simulink model "PubIfDecisionTOS_MDL"  (R2020b)
settings: configuration reference "DspaceConfig" (kept outside this file)
PostLoadFcn:
  | if any(exist('dsrtsu_mdlpostloadfcn', 'file') ~= 0), dsrtsu_mdlpostloadfcn('Execute', bdroot); end
InitFcn:
  | , if any(exist('dsmpb_private', 'file') ~= 0), dsmpb_private('dsmpb_mdlclblib', 'Init', bdroot); end,
undefined symbols (not defined in the file or in its folder): C_TOS_ACCEgoRAxletoFbumplength_m, C_TOS_ACCTargetFront_Flag, C_TOS_AEBJAPedObjDxThre_Val, C_TOS_AEBJAPedObjDyThre_Val, C_TOS_AEBJATargetSize_Val, C_TOS_AEBJAVehObjDxThre_Val, C_TOS_AEBJAVehObjDyThre_Val, C_TOS_AEBJuncPedTargetSize_Val, C_TOS_AEBLatObjDxThre_Val, C_TOS_AEBLatPedDyThre_Val, C_TOS_AEBLatTargetSize_Val, C_TOS_AEBLongTargetInEgoFront_Flag, C_TOS_axAbsGround_Parameter, C_TOS_CameraConfirmedFlag, C_TOS_CNsubjWidth, C_TOS_CurrentLaneCoreMinWidth_Val, C_TOS_CutInProb_Val_Zero, C_TOS_CutOutProb_Val_Zero, C_TOS_D2R_Val, C_TOS_DefaultValueObjectToCenterLine_dy, C_TOS_EgoCarWidth_Val, C_TOS_EgoDxRefPoint_m, C_TOS_EgoRAxletoFbumplength_m, C_TOS_HalfWidthVehicle_Con, C_TOS_HWA_CurrentLaneFlag, C_TOS_HWA_LeftLaneFlag, C_TOS_HWA_MovingDir_Vaild, C_TOS_HWA_MovState_Vaild, C_TOS_HWA_RightLaneFlag, C_TOS_LaneLineCourseErrorFront, C_TOS_LaneLineCourseErrorRear, C_TOS_MotorbikeDefaultWidth_m, C_TOS_NumberOfEffectiveTargets, C_TOS_Obj_Age_Val, C_TOS_Objdx_Constraint_Val, C_TOS_ObjectDefaultWidth_m, C_TOS_ObjInCurrentLane_Val, C_TOS_ObjInCurrentLaneValid, C_TOS_ObjInLeftLaneValid, C_TOS_ObjInRightLaneValid, C_TOS_ObjNotInCurrentLane_Val, C_TOS_ObjNotREElementType, C_TOS_ObjPredictDis_dy_ConstantVal_Zeros, C_TOS_ObjToCenterLine_ConstantVal_Zeros, C_TOS_OFMObjIDInvilad_Val, C_TOS_PIL_LatDisCons_Val_zero, C_TOS_PIL_ObjectCutInFlag_b, C_TOS_PIL_ObjectCutOutFlag_b, C_TOS_PIL_ObjLaneProb_al_Val, C_TOS_PP_ObjFusType_FC_Confirm_b, C_TOS_PP_ObjFusType_FC_FR_Confirm_b, C_TOS_PP_ObjFusType_FR_Confirm_b, C_TOS_RE_80BoolDefault_Val, C_TOS_RE_80Single181Default_Val, C_TOS_RE_80Single255Default_Val, C_TOS_RE_80Uint8Default_Val, C_TOS_RE_D2R, C_TOS_RE_D_180_Val, C_TOS_RE_InvalidObjectID_Val, C_TOS_RE_InvalidTargetChainDir_Val ... (+142)
libraries: simulink x1650, TOS_LIB x361, canfdmsglib x14
(part 68 of 69)

== stateflow chart PubIfDecisionTOS_MDL/TOS_20201112/TOS_2012080320/TOS/AEB/TOS_AEBLatCro_20201208/AEBLatTrgInfor/TOS_AEBLatCro ==
  (default) -> (junction 57) : {i=uint8(1);}
  (junction 57) -> (junction 61) [order 1] : [i<=C_TOS_AEBLatTargetSize_Val]
  (junction 64) -> (junction 57) : {i=i+uint8(1);}
  (junction 57) -> (junction 47) [order 2]
  (junction 61) -> (junction 64) : {
      | TOS_AEBLatTargetBus(i).FusionType= uint8(0);
      | TOS_AEBLatTargetBus(i).ObjectID= uint8(0);
      | TOS_AEBLatTargetBus(i).ObjectType= uint8(0);
      | TOS_AEBLatTargetBus(i).ObjectTypeCameraConfirmed= false;
      | TOS_AEBLatTargetBus(i).ObjectLength=single(0);
      | TOS_AEBLatTargetBus(i).ObjectWidth= single(0);
      | TOS_AEBLatTargetBus(i).ObjectHight= single(0);
      | TOS_AEBLatTargetBus(i).ObjectYawAngle= single(0);
      | TOS_AEBLatTargetBus(i).ObjectAzimuthAngle= single(0);
      | TOS_AEBLatTargetBus(i).ObjectMovingState= uint8(0);
      | TOS_AEBLatTargetBus(i).ObjectMovingOrientation=uint8(0);
      | TOS_AEBLatTargetBus(i).dxFisrtDetection= single(0);
      | TOS_AEBLatTargetBus(i).dyFisrtDetection= single(0);
      | TOS_AEBLatTargetBus(i).dx= single(0);
      | TOS_AEBLatTargetBus(i).dy= single(0);
      | TOS_AEBLatTargetBus(i).dz= single(0);
      | TOS_AEBLatTargetBus(i).vx= single(0);
      | TOS_AEBLatTargetBus(i).vy= single(0);
      | TOS_AEBLatTargetBus(i).ax= single(0);
      | TOS_AEBLatTargetBus(i).ay= single(0);
      | TOS_AEBLatTargetBus(i).dxVariance= single(0);
      | TOS_AEBLatTargetBus(i).dyVariance= single(0);
      | TOS_AEBLatTargetBus(i).vxVariance= single(0);
      | TOS_AEBLatTargetBus(i).vyVariance= single(0);
      | TOS_AEBLatTargetBus(i).axVariance= single(0);
      | TOS_AEBLatTargetBus(i).ayVariance= single(0);
      | TOS_AEBLatTargetBus(i).ObjectLengthVar= single(0);
      | TOS_AEBLatTargetBus(i).ObjectWidthVar= single(0);
      | TOS_AEBLatTargetBus(i).ObjectYawAngleVar= single(0);
      | TOS_AEBLatTargetBus(i).ObjectTypeProb= single(0);
      | TOS_AEBLatTargetBus(i).ObjectMovingStateProb= single(0);
      | TOS_AEBLatTargetBus(i).ObjectMovingOrientationProb= single(0);
      | TOS_AEBLatTargetBus(i).ObjectExistProb= single(0);
      | TOS_AEBLatTargetBus(i).ObjectIsObstacleProb= single(0);
      | TOS_AEBLatTargetBus(i).ObjectRCS= single(0);
      | TOS_AEBLatTargetBus(i).ObjectMeasurementStatus= single(0);
      | TOS_AEBLatTargetBus(i).ObjectLifeCycle= uint16(0);
      | TOS_AEBLatTargetBus(i).ObjUpdate= false;
      | }
  (junction 47) -> (junction 50) : {i=uint8(1);
      | j=uint8(1);}
  (junction 50) -> (junction 60) [order 1] : [i<=C_TOS_AEBLatTargetSize_Val]
  (junction 48) -> (junction 50) : {i=i+uint8(1);}
  (junction 50) -> (junction 63) [order 2]
  (junction 60) -> (junction 62)
  (junction 62) -> (junction 52) [order 1] : [TOS_AEBLatTargetIndex(i)~=uint8(0)]
  (junction 62) -> (junction 48) [order 2]
  (junction 52) -> (junction 65) : {
      | TargetIndex = TOS_AEBLatTargetIndex(i);
      | TOS_AEBLatTargetBus(j).FusionType=OFM_SignalVerification.Object_Fus_Type(TargetIndex);
      | TOS_AEBLatTargetBus(j).ObjectID=OFM_SignalVerification.Object_ID(TargetIndex);
      | TOS_AEBLatTargetBus(j).ObjectType=AEBLat_TargetObjectType(i);
      | TOS_AEBLatTargetBus(j).ObjectTypeCameraConfirmed=TOS_AddAttributes.PP_CamareConfirmSignalProcessing(TargetIndex);
      | TOS_AEBLatTargetBus(j).ObjectLength=OFM_SignalVerification.Object_Length(TargetIndex);
      | TOS_AEBLatTargetBus(j).ObjectWidth=OFM_SignalVerification.Object_Width(TargetIndex);
      | TOS_AEBLatTargetBus(j).ObjectHight=OFM_SignalVerification.Object_Hight(TargetIndex);
      | TOS_AEBLatTargetBus(j).ObjectYawAngle=OFM_SignalVerification.Object_HeadingAngle(TargetIndex);
      | TOS_AEBLatTargetBus(j).ObjectAzimuthAngle=OFM_SignalVerification.Object_YawAngle(TargetIndex);
      | TOS_AEBLatTargetBus(j).ObjectMovingState=TOS_AddAttributes.PP_MovingState_AEB_SignalProcessing(TargetIndex);
      | TOS_AEBLatTargetBus(j).ObjectMovingOrientation=uint8(3);%Crossing
      | TOS_AEBLatTargetBus(j).dxFisrtDetection=TOS_AddAttributes.PP_ObjFirstDetect_Dx(TargetIndex);
      | TOS_AEBLatTargetBus(j).dyFisrtDetection=TOS_AddAttributes.PP_ObjFirstDetect_Dy(TargetIndex);
      | TOS_AEBLatTargetBus(j).dx=OFM_SignalVerification.Object_DX(TargetIndex);
      | TOS_AEBLatTargetBus(j).dy=OFM_SignalVerification.Object_DY(TargetIndex);
      | TOS_AEBLatTargetBus(j).dz= single(0);
      | TOS_AEBLatTargetBus(j).vx=OFM_SignalVerification.Object_VX(TargetIndex);
      | TOS_AEBLatTargetBus(j).vy=OFM_SignalVerification.Object_VY(TargetIndex);
      | TOS_AEBLatTargetBus(j).ax=OFM_SignalVerification.Object_AX(TargetIndex);
      | TOS_AEBLatTargetBus(j).ay=OFM_SignalVerification.Object_AY(TargetIndex);
      | TOS_AEBLatTargetBus(j).dxVariance=OFM_SignalVerification.Object_Std_DX(TargetIndex);
      | TOS_AEBLatTargetBus(j).dyVariance=OFM_SignalVerification.Object_Std_DY(TargetIndex);
      | TOS_AEBLatTargetBus(j).vxVariance=OFM_SignalVerification.Object_Std_VX(TargetIndex);
      | TOS_AEBLatTargetBus(j).vyVariance=OFM_SignalVerification.Object_Std_VY(TargetIndex);
      | TOS_AEBLatTargetBus(j).axVariance=OFM_SignalVerification.Object_Std_AX(TargetIndex);
      | TOS_AEBLatTargetBus(j).ayVariance=OFM_SignalVerification.Object_Std_AY(TargetIndex);
      | TOS_AEBLatTargetBus(j).ObjectLengthVar=OFM_SignalVerification.Object_Std_Length(TargetIndex);
      | TOS_AEBLatTargetBus(j).ObjectWidthVar=OFM_SignalVerification.Object_Std_Width(TargetIndex);
      | TOS_AEBLatTargetBus(j).ObjectYawAngleVar=OFM_SignalVerification.Object_Std_HeadingAngle(TargetIndex);
      | TOS_AEBLatTargetBus(j).ObjectTypeProb=OFM_SignalVerification.Object_Type_Prob(TargetIndex);
      | TOS_AEBLatTargetBus(j).ObjectMovingStateProb= single(0);
      | TOS_AEBLatTargetBus(j).ObjectMovingOrientationProb= single(0);
      | TOS_AEBLatTargetBus(j).ObjectExistProb=OFM_SignalVerification.Object_ExistProb(TargetIndex);
      | TOS_AEBLatTargetBus(j).ObjectIsObstacleProb=OFM_SignalVerification.Object_ObstacleProb(TargetIndex);
      | TOS_AEBLatTargetBus(j).ObjectRCS= single(0);
      | TOS_AEBLatTargetBus(j).ObjectMeasurementStatus= single(0);
      | TOS_AEBLatTargetBus(j).ObjectLifeCycle=OFM_SignalVerification.Object_Age(TargetIndex);
      | TOS_AEBLatTargetBus(j).ObjUpdate= false;
      | j=j+uint8(1);
      | }
  (junction 65) -> (junction 48)
  data: TOS_AddAttributes input Bus: TOS_AddAttributes_BUS; OFM_SignalVerification input Bus: OFM_OBJ_BUS; AEBLat_TargetObjectType input; TOS_AEBLatTargetIndex input uint8 size=10; TOS_AEBLatTargetBus output Bus: TOS_AEB_LATOBJ_BUS size=10; C_TOS_AEBLatTargetSize_Val parameter; TargetIndex local uint8; i local uint8; j local uint8

== stateflow chart PubIfDecisionTOS_MDL/TOS_20201112/TOS_2012080320/TOS/ACC/TOS_ACCCurrentLane/ACC_CurrentLane_Target/TOS_ACC_P0/ACC_P0_Targe/ACC_P0_Targe/TOS_ACC_TargetMovingDirConfirm/TOS_ACC_TargetMovingDirConfirm_V2011170316(备份)/Subsystem/TOS_ObjMovStateCfmFlow ==
  note: TOS_ObjMovStateCfm Coding:
      | 0: Object default moving state
      | 1：Object had been moving
      | 2: Object had been Stopped
  (default) -> (junction 1)
  (junction 1) -> (junction 3) [order 1] : [Target_ID_K1 ~=C_TOS_OFMObjIDInvilad_Val&&...
      | Target_ID_K2 ~= C_TOS_OFMObjIDInvilad_Val]
  (junction 1) -> (junction 38) [order 2] : {
      |   TOS_ObjMovStateCfm = uint8(0);
      | }
  (junction 3) -> (junction 5)
  (junction 5) -> (junction 7) [order 1] : [Target_ID_K1 ==Target_ID_K2]
  (junction 5) -> (junction 35) [order 2] : {
      |   TOS_ObjMovStateCfm =uint8(0);
      | }
  (junction 7) -> (junction 9)
  (junction 9) -> (junction 11) [order 1] : [ObjectID ==Target_ID_K1]
  (junction 9) -> (junction 29) [order 2] : {
      |   TOS_ObjMovStateCfm = uint8(0);
      | }
  (junction 11) -> (junction 13)
  (junction 13) -> (junction 15) [order 1] : [Target_MovState_K2 == ObjectMovingState_E.Moving&&...
      | Target_MovState_K1 == ObjectMovingState_E.Moving||...
      |   TOS_ObjMovStateCfm == uint8(1)]
  (junction 13) -> (junction 52) [order 2]
  (junction 15) -> (junction 58) : {
      |   TOS_ObjMovStateCfm = uint8(1);
      | }
  (junction 52) -> (junction 23) [order 1] : [Target_MovState_K2 == ObjectMovingState_E.Stopped&&...
      | Target_MovState_K1 == ObjectMovingState_E.Stopped||...
      |   TOS_ObjMovStateCfm == uint8(2)]
  (junction 52) -> (junction 27) [order 2] : {
      |   TOS_ObjMovStateCfm = uint8(0);
      | }
  (junction 23) -> (junction 54) : {
      |   TOS_ObjMovStateCfm = uint8(2);
      | }
  (junction 35) -> (junction 38)
  (junction 29) -> (junction 35)
  (junction 27) -> (junction 29)
  (junction 54) -> (junction 27)
  (junction 58) -> (junction 54)
  (junction 38) -> (junction 41)
  data: Target_ID_K1 input uint8; Target_ID_K2 input uint8; Target_MovState_K1 input Enum: ObjectMovingState_E; Target_MovState_K2 input Enum: ObjectMovingState_E; ObjMovState input Enum: OFM_OBJ_MOVINGSTATE_E; ObjectID input uint8; TOS_ObjMovStateCfm output uint8; C_TOS_OFMObjIDInvilad_Val parameter uint8

== stateflow chart PubIfDecisionTOS_MDL/TOS_20201112/TOS_2012080320/TOS/AEB/TOS_AEBLatCro_20201208/AEBLat_Object_Condition/AEBLat_TargetCondition/TOS_AEBLat_TargetsDx/Chart ==
  state AEBLatSameTargetIDJudge [function]
    (default) -> (junction 70) : {
        | i = uint8(1);
        | AEBLat_SameTarget = false;
        | }
    (junction 70) -> (junction 81) [order 1] : [i<=C_TOS_AEBLatTargetSize_Val]
    (junction 86) -> (junction 70)
    (junction 70) -> (junction 83) [order 2]
    (junction 81) -> (junction 77)
    (junction 77) -> (junction 78) [order 1] : [AEBLat_Target_ObjectID_K1(i) == Object_ID]
    (junction 77) -> (junction 74) [order 2] : %donothing
    (junction 78) -> (junction 72) : {
        | AEBLat_SameTarget = true;
        | }
    (junction 72) -> (junction 74)
    (junction 74) -> (junction 86) : {i = i+1;}
  (default) -> (junction 1)
  (junction 1) -> (junction 3) [order 1] : [AEBLat_TargetCondition == true]
  (junction 1) -> (junction 97) [order 2] : {
      | TOS_AEBLat_TargetsDx = single(255);
      | }
  (junction 3) -> (junction 88) : {
      | AEBLatSameTargetIDJudge();
      | }
  (junction 88) -> (junction 124) [order 1] : [AEBLat_SameTarget == false]
  (junction 88) -> (junction 94) [order 2] : {
      | TOS_AEBLat_TargetsDx = Object_Dx;
      | }
  (junction 124) -> (junction 114)
  (junction 114) -> (junction 117) [order 1] : [abs(Object_Vy) > P_TOS_CrossingTargetVyvThre_val &&...
      | abs(psiDtOpt) < P_TOS_AEBLatTargetEgoYawRateThre_val]
  (junction 114) -> (junction 118) [order 2] : {
      | TOS_AEBLat_TargetsDx = single(255);
      | }
  (junction 117) -> (junction 112) : {
      | TOS_AEBLat_TargetsDx = Object_Dx;
      | }
  (junction 112) -> (junction 118)
  (junction 118) -> (junction 125)
  (junction 94) -> (junction 97)
  (junction 125) -> (junction 94)
  (junction 97) -> (junction 100)
  data: AEBLat_TargetCondition input boolean; Object_ID input uint8; psiDtOpt input single; AEBLat_Target_ObjectID_K1 input uint8 size=10; Object_Vy input single; TOS_AEBLat_TargetsDx output single size=1; Object_Dx input single; AEBLat_SameTarget local boolean size=1 =false; P_TOS_CrossingTargetVyvThre_val parameter; P_TOS_AEBLatTargetEgoYawRateThre_val parameter; C_TOS_AEBLatTargetSize_Val parameter

== stateflow chart PubIfDecisionTOS_MDL/TOS_20201112/TOS_2012080320/TOS/AEB/TOS_AEBLatCro_20201208/AEBLat_Object_Condition2/AEBLat_TargetCondition/TOS_AEBLat_TargetsDx/Chart ==
  state AEBLatSameTargetIDJudge [function]
    (default) -> (junction 70) : {
        | i = uint8(1);
        | AEBLat_SameTarget = false;
        | }
    (junction 70) -> (junction 81) [order 1] : [i<=C_TOS_AEBLatTargetSize_Val]
    (junction 86) -> (junction 70)
    (junction 70) -> (junction 83) [order 2]
    (junction 81) -> (junction 77)
    (junction 77) -> (junction 78) [order 1] : [AEBLat_Target_ObjectID_K1(i) == Object_ID]
    (junction 77) -> (junction 74) [order 2] : %donothing
    (junction 78) -> (junction 72) : {
        | AEBLat_SameTarget = true;
        | }
    (junction 72) -> (junction 74)
    (junction 74) -> (junction 86) : {i = i+1;}
  (default) -> (junction 1)
  (junction 1) -> (junction 3) [order 1] : [AEBLat_TargetCondition == true]
  (junction 1) -> (junction 97) [order 2] : {
      | TOS_AEBLat_TargetsDx = single(255);
      | }
  (junction 3) -> (junction 88) : {
      | AEBLatSameTargetIDJudge();
      | }
  (junction 88) -> (junction 124) [order 1] : [AEBLat_SameTarget == false]
  (junction 88) -> (junction 94) [order 2] : {
      | TOS_AEBLat_TargetsDx = Object_Dx;
      | }
  (junction 124) -> (junction 114)
  (junction 114) -> (junction 117) [order 1] : [abs(Object_Vy) > P_TOS_CrossingTargetVyvThre_val &&...
      | abs(psiDtOpt) < P_TOS_AEBLatTargetEgoYawRateThre_val]
  (junction 114) -> (junction 118) [order 2] : {
      | TOS_AEBLat_TargetsDx = single(255);
      | }
  (junction 117) -> (junction 112) : {
      | TOS_AEBLat_TargetsDx = Object_Dx;
      | }
  (junction 112) -> (junction 118)
  (junction 118) -> (junction 125)
  (junction 94) -> (junction 97)
  (junction 125) -> (junction 94)
  (junction 97) -> (junction 100)
  data: AEBLat_TargetCondition input boolean; Object_ID input uint8; psiDtOpt input single; AEBLat_Target_ObjectID_K1 input uint8 size=10; Object_Vy input single; TOS_AEBLat_TargetsDx output single size=1; Object_Dx input single; AEBLat_SameTarget local boolean size=1 =false; P_TOS_CrossingTargetVyvThre_val parameter; P_TOS_AEBLatTargetEgoYawRateThre_val parameter; C_TOS_AEBLatTargetSize_Val parameter

== matlab function PubIfDecisionTOS_MDL/TOS_20201112/TOS_2012080320/TOS/AEB/TOS_AEBLatCro_20201208/AEBLat_TargetIndex/MATLAB Function ==
  data: Object_Num input; Object_Dx input; ObjDxIndex output
function ObjDxIndex  = fcn(Object_Num, Object_Dx)
ObjNum=int32(80);
ObjDxIndex=uint8(zeros(ObjNum,1));

DxDy=Object_Dx;
MidIndex=int32(1):int32(1):ObjNum;

for i=1:Object_Num
    ObjDxIndex(i)=MidIndex(i);
    t_dis=DxDy(i);
    if i<Object_Num-1
        for j=(i+1):Object_Num
            if DxDy(j)<t_dis
                temp_index=ObjDxIndex(i);
                temp_dis=t_dis;
                
                ObjDxIndex(i)=MidIndex(j);
                DxDy(i)=DxDy(j);
                t_dis=DxDy(j);
                MidIndex(j)=temp_index;
                DxDy(j)=temp_dis;
            end
            
            if DxDy(i) >= single(250)     
                ObjDxIndex(i)=uint8(0); 
            end           
   
        end
    else
        if i~=Object_Num
            if DxDy(Object_Num)<t_dis
                temp_index=ObjDxIndex(i);
                temp_dis=t_dis;
                ObjDxIndex(i)=MidIndex(Object_Num);
                DxDy(i)=DxDy(Object_Num);
                MidIndex(Object_Num)=temp_index;
                DxDy(Object_Num)=temp_dis;
            else
                MidIndex(Object_Num)=MidIndex(Object_Num);
                DxDy(Object_Num)=DxDy(Object_Num);
            end
            
            if DxDy(i) >= single(250)     
                ObjDxIndex(i)=uint8(0); 
            end       
            
        end
    end

end

== stateflow chart PubIfDecisionTOS_MDL/TOS_20201112/TOS_2012080320/TOS/AEB/TOS_AEBLong/AEBLongTargetInfor/TOS_AEBLong ==
  (default) -> (junction 1)
  (junction 1) -> (junction 3) [order 1] : [TOS_AEBLongTargetIndex ~= uint8(0)]
  (junction 1) -> (junction 7) [order 2] : {TOS_AEBLongTargetBus.FusionType= uint8(0);
      | TOS_AEBLongTargetBus.ObjectID= uint8(0);
      | TOS_AEBLongTargetBus.ObjectType= uint8(0);
      | TOS_AEBLongTargetBus.ObjectTypeCameraConfirmed= boolean(0);
      | TOS_AEBLongTargetBus.ObjectLength= single(0);
      | TOS_AEBLongTargetBus.ObjectWidth= single(0);
      | TOS_AEBLongTargetBus.ObjectHight= single(0);
      | TOS_AEBLongTargetBus.ObjectYawAngle= single(0);
      | TOS_AEBLongTargetBus.ObjectAzimuthAngle= single(0);
      | TOS_AEBLongTargetBus.ObjectMovingState= uint8(0);
      | TOS_AEBLongTargetBus.ObjectMovingOrientation=uint8(0);
      | TOS_AEBLongTargetBus.dxFisrtDetection= single(0);
      | TOS_AEBLongTargetBus.dyFisrtDetection= single(0);
      | TOS_AEBLongTargetBus.dx= single(0);
      | TOS_AEBLongTargetBus.dy= single(0);
      | TOS_AEBLongTargetBus.dz= single(0);
      | TOS_AEBLongTargetBus.vx= single(0);
      | TOS_AEBLongTargetBus.vy= single(0);
      | TOS_AEBLongTargetBus.ax= single(0);
      | TOS_AEBLongTargetBus.ay= single(0);
      | TOS_AEBLongTargetBus.dxVariance= single(0);
      | TOS_AEBLongTargetBus.dyVariance= single(0);
      | TOS_AEBLongTargetBus.vxVariance= single(0);
      | TOS_AEBLongTargetBus.vyVariance= single(0);
      | TOS_AEBLongTargetBus.axVariance= single(0);
      | TOS_AEBLongTargetBus.ayVariance= single(0);
      | TOS_AEBLongTargetBus.ObjectLengthVar= single(0);
      | TOS_AEBLongTargetBus.ObjectWidthVar= single(0);
      | TOS_AEBLongTargetBus.ObjectYawAngleVar= single(0);
      | TOS_AEBLongTargetBus.ObjectTypeProb= single(0);
      | TOS_AEBLongTargetBus.ObjectMovingStateProb= single(0);
      | TOS_AEBLongTargetBus.ObjectMovingOrientationProb= single(0);
      | TOS_AEBLongTargetBus.ObjectExistProb= single(0);
      | TOS_AEBLongTargetBus.ObjectIsObstacleProb= single(0);
      | TOS_AEBLongTargetBus.ObjectRCS= single(0);
      | TOS_AEBLongTargetBus.ObjectMeasurementStatus= single(0);
      | TOS_AEBLongTargetBus.ObjectLifeCycle= single(0);
      | TOS_AEBLongTargetBus.dyObject2Center= single(0);
      | TOS_AEBLongTargetBus.dyEgo2Center= single(0);
      | TOS_AEBLongTargetBus.ObjUpdate=false;
      | }
  (junction 3) -> (junction 5) : {
      | TOS_AEBLongTargetBus.FusionType=OFM_SignalVerification.Object_Fus_Type[TOS_AEBLongTargetIndex- uint8(1)];
      | TOS_AEBLongTargetBus.ObjectID=OFM_SignalVerification.Object_ID[TOS_AEBLongTargetIndex-uint8(1)];
      | TOS_AEBLongTargetBus.ObjectType=OFM_SignalVerification.Object_Type[TOS_AEBLongTargetIndex- uint8(1)];
      | TOS_AEBLongTargetBus.ObjectTypeCameraConfirmed=TOS_AddAttributes.PP_CamareConfirmSignalProcessing[TOS_AEBLongTargetIndex-uint8(1)];
      | TOS_AEBLongTargetBus.ObjectLength=OFM_SignalVerification.Object_Length[TOS_AEBLongTargetIndex-uint8(1)];
      | TOS_AEBLongTargetBus.ObjectWidth=OFM_SignalVerification.Object_Width[TOS_AEBLongTargetIndex-uint8(1)];
      | TOS_AEBLongTargetBus.ObjectHight=OFM_SignalVerification.Object_Hight[TOS_AEBLongTargetIndex-uint8(1)];
      | TOS_AEBLongTargetBus.ObjectYawAngle=OFM_SignalVerification.Object_HeadingAngle[TOS_AEBLongTargetIndex-uint8(1)];
      | TOS_AEBLongTargetBus.ObjectAzimuthAngle=OFM_SignalVerification.Object_YawAngle[TOS_AEBLongTargetIndex-uint8(1)];
      | TOS_AEBLongTargetBus.ObjectMovingState = TOS_AddAttributes.PP_MovingState_AEB_SignalProcessing[TOS_AEBLongTargetIndex-uint8(1)];
      | TOS_AEBLongTargetBus.ObjectMovingOrientation=TOS_AEBLongTargetMovingDir;
      | TOS_AEBLongTargetBus.dxFisrtDetection=TOS_AddAttributes.PP_ObjFirstDetect_Dx[TOS_AEBLongTargetIndex-uint8(1)];
      | TOS_AEBLongTargetBus.dyFisrtDetection=TOS_AddAttributes.PP_ObjFirstDetect_Dy[TOS_AEBLongTargetIndex-uint8(1)];
      | TOS_AEBLongTargetBus.dx=OFM_SignalVerification.Object_DX[TOS_AEBLongTargetIndex-uint8(1)];
      | TOS_AEBLongTargetBus.dy=OFM_SignalVerification.Object_DY[TOS_AEBLongTargetIndex-uint8(1)];
      | TOS_AEBLongTargetBus.dz= single(0);
      | TOS_AEBLongTargetBus.vx=OFM_SignalVerification.Object_VX[TOS_AEBLongTargetIndex-uint8(1)];
      | TOS_AEBLongTargetBus.vy=OFM_SignalVerification.Object_VY[TOS_AEBLongTargetIndex-uint8(1)];
      | TOS_AEBLongTargetBus.ax=OFM_SignalVerification.Object_AX[TOS_AEBLongTargetIndex-uint8(1)];
      | TOS_AEBLongTargetBus.ay=OFM_SignalVerification.Object_AY[TOS_AEBLongTargetIndex-uint8(1)];
      | TOS_AEBLongTargetBus.dxVariance=OFM_SignalVerification.Object_Std_DX[TOS_AEBLongTargetIndex-uint8(1)];
      | TOS_AEBLongTargetBus.dyVariance=OFM_SignalVerification.Object_Std_DY[TOS_AEBLongTargetIndex-uint8(1)];
      | TOS_AEBLongTargetBus.vxVariance=OFM_SignalVerification.Object_Std_VX[TOS_AEBLongTargetIndex-uint8(1)];
      | TOS_AEBLongTargetBus.vyVariance=OFM_SignalVerification.Object_Std_VY[TOS_AEBLongTargetIndex-uint8(1)];
      | TOS_AEBLongTargetBus.axVariance=OFM_SignalVerification.Object_Std_AX[TOS_AEBLongTargetIndex-uint8(1)];
      | TOS_AEBLongTargetBus.ayVariance=OFM_SignalVerification.Object_Std_AY[TOS_AEBLongTargetIndex-uint8(1)];
      | TOS_AEBLongTargetBus.ObjectLengthVar=OFM_SignalVerification.Object_Std_Length[TOS_AEBLongTargetIndex-uint8(1)];
      | TOS_AEBLongTargetBus.ObjectWidthVar=OFM_SignalVerification.Object_Std_Width[TOS_AEBLongTargetIndex-uint8(1)];
      | TOS_AEBLongTargetBus.ObjectYawAngleVar=OFM_SignalVerification.Object_Std_HeadingAngle[TOS_AEBLongTargetIndex-uint8(1)];
      | TOS_AEBLongTargetBus.ObjectTypeProb=OFM_SignalVerification.Object_Type_Prob[TOS_AEBLongTargetIndex-uint8(1)];
      | TOS_AEBLongTargetBus.ObjectMovingStateProb= single(0);
      | TOS_AEBLongTargetBus.ObjectMovingOrientationProb= single(0);
      | TOS_AEBLongTargetBus.ObjectExistProb=OFM_SignalVerification.Object_ExistProb[TOS_AEBLongTargetIndex-uint8(1)];
      | TOS_AEBLongTargetBus.ObjectIsObstacleProb=OFM_SignalVerification.Object_ObstacleProb[TOS_AEBLongTargetIndex-uint8(1)];
      | TOS_AEBLongTargetBus.ObjectRCS= single(0);
      | TOS_AEBLongTargetBus.ObjectMeasurementStatus= single(0);
      | TOS_AEBLongTargetBus.ObjectLifeCycle=OFM_SignalVerification.Object_Age[TOS_AEBLongTargetIndex-uint8(1)];
      | TOS_AEBLongTargetBus.dyObject2Center=TOS_AddAttributes.PP_ObjectToCenterLine_dy[TOS_AEBLongTargetIndex-uint8(1)];
      | TOS_AEBLongTargetBus.dyEgo2Center=TOS_AddAttributes.PP_EgoVehCenterLine_dy;
      | TOS_AEBLongTargetBus.ObjUpdate=false;
      | }
  (junction 5) -> (junction 7)
  (junction 7) -> (junction 11)
  data: OFM_SignalVerification input Bus: OFM_OBJ_BUS; TOS_AddAttributes input Bus: TOS_AddAttributes_BUS; TOS_AEBLongTargetMovingDir input uint8; TOS_AEBLongTargetIndex input uint8; TOS_AEBLongTargetBus output Bus: TOS_AEB_LONOBJ_BUS

== stateflow chart PubIfDecisionTOS_MDL/TOS_20201112/TOS_2012080320/TOS/AEB/TOS_AEBLong/AEBLongTargetInfor/TOS_AEBLong1 ==
  (default) -> (junction 1)
  (junction 1) -> (junction 3) [order 1] : [TOS_AEBLongTargetIndex ~= uint8(0)]
  (junction 1) -> (junction 7) [order 2] : {TOS_AEBLongTargetBus.FusionType= uint8(0);
      | TOS_AEBLongTargetBus.ObjectID= uint8(0);
      | TOS_AEBLongTargetBus.ObjectType= uint8(0);
      | TOS_AEBLongTargetBus.ObjectTypeCameraConfirmed= boolean(0);
      | TOS_AEBLongTargetBus.ObjectLength= single(0);
      | TOS_AEBLongTargetBus.ObjectWidth= single(0);
      | TOS_AEBLongTargetBus.ObjectHight= single(0);
      | TOS_AEBLongTargetBus.ObjectYawAngle= single(0);
      | TOS_AEBLongTargetBus.ObjectAzimuthAngle= single(0);
      | TOS_AEBLongTargetBus.ObjectMovingState= uint8(0);
      | TOS_AEBLongTargetBus.ObjectMovingOrientation=uint8(0);
      | TOS_AEBLongTargetBus.dxFisrtDetection= single(0);
      | TOS_AEBLongTargetBus.dyFisrtDetection= single(0);
      | TOS_AEBLongTargetBus.dx= single(0);
      | TOS_AEBLongTargetBus.dy= single(0);
      | TOS_AEBLongTargetBus.dz= single(0);
      | TOS_AEBLongTargetBus.vx= single(0);
      | TOS_AEBLongTargetBus.vy= single(0);
      | TOS_AEBLongTargetBus.ax= single(0);
      | TOS_AEBLongTargetBus.ay= single(0);
      | TOS_AEBLongTargetBus.dxVariance= single(0);
      | TOS_AEBLongTargetBus.dyVariance= single(0);
      | TOS_AEBLongTargetBus.vxVariance= single(0);
      | TOS_AEBLongTargetBus.vyVariance= single(0);
      | TOS_AEBLongTargetBus.axVariance= single(0);
      | TOS_AEBLongTargetBus.ayVariance= single(0);
      | TOS_AEBLongTargetBus.ObjectLengthVar= single(0);
      | TOS_AEBLongTargetBus.ObjectWidthVar= single(0);
      | TOS_AEBLongTargetBus.ObjectYawAngleVar= single(0);
      | TOS_AEBLongTargetBus.ObjectTypeProb= single(0);
      | TOS_AEBLongTargetBus.ObjectMovingStateProb= single(0);
      | TOS_AEBLongTargetBus.ObjectMovingOrientationProb= single(0);
      | TOS_AEBLongTargetBus.ObjectExistProb= single(0);
      | TOS_AEBLongTargetBus.ObjectIsObstacleProb= single(0);
      | TOS_AEBLongTargetBus.ObjectRCS= single(0);
      | TOS_AEBLongTargetBus.ObjectMeasurementStatus= single(0);
      | TOS_AEBLongTargetBus.ObjectLifeCycle= single(0);
      | TOS_AEBLongTargetBus.dyObject2Center= single(0);
      | TOS_AEBLongTargetBus.dyEgo2Center= single(0);
      | TOS_AEBLongTargetBus.ObjUpdate=false;
      | }
  (junction 3) -> (junction 5) : {
      | TOS_AEBLongTargetBus.FusionType                  =OFM_SignalVerification.Object_Fus_Type[TOS_AEBLongTargetIndex- uint8(1)];
      | TOS_AEBLongTargetBus.ObjectID                      =OFM_SignalVerification.Object_ID[TOS_AEBLongTargetIndex-uint8(1)];
      | TOS_AEBLongTargetBus.ObjectType                 =OFM_SignalVerification.Object_Type[TOS_AEBLongTargetIndex- uint8(1)];
      | TOS_AEBLongTargetBus.ObjectTypeCameraConfirmed             =TOS_AddAttributes.PP_CamareConfirmSignalProcessing[TOS_AEBLongTargetIndex-uint8(1)];
      | TOS_AEBLongTargetBus.ObjectLength               =OFM_SignalVerification.Object_Length[TOS_AEBLongTargetIndex-uint8(1)];
      | TOS_AEBLongTargetBus.ObjectWidth                 =OFM_SignalVerification.Object_Width[TOS_AEBLongTargetIndex-uint8(1)];
      | TOS_AEBLongTargetBus.ObjectHight                  =OFM_SignalVerification.Object_Hight[TOS_AEBLongTargetIndex-uint8(1)];
      | TOS_AEBLongTargetBus.ObjectYawAngle           =OFM_SignalVerification.Object_HeadingAngle[TOS_AEBLongTargetIndex-uint8(1)];
      | TOS_AEBLongTargetBus.ObjectAzimuthAngle     =OFM_SignalVerification.Object_YawAngle[TOS_AEBLongTargetIndex-uint8(1)];
      | TOS_AEBLongTargetBus.ObjectMovingState       =TOS_AEBLongTargetMovingDir;
      | TOS_AEBLongTargetBus.ObjectMovingOrientation                =TOS_AddAttributes.PP_ObjMovingDirSignalProcessing[TOS_AEBLongTargetIndex-uint8(1)];
      | TOS_AEBLongTargetBus.dxFisrtDetection            =TOS_AddAttributes.PP_ObjFirstDetect_Dx[TOS_AEBLongTargetIndex-uint8(1)];
      | TOS_AEBLongTargetBus.dyFisrtDetection             =TOS_AddAttributes.PP_ObjFirstDetect_Dy[TOS_AEBLongTargetIndex-uint8(1)];
      | TOS_AEBLongTargetBus.dx                                   =OFM_SignalVerification.Object_DX[TOS_AEBLongTargetIndex-uint8(1)];
      | TOS_AEBLongTargetBus.dy                                   =OFM_SignalVerification.Object_DY[TOS_AEBLongTargetIndex-uint8(1)];
      | TOS_AEBLongTargetBus.dz= single(0);
      | TOS_AEBLongTargetBus.vx=OFM_SignalVerification.Object_VX[TOS_AEBLongTargetIndex-uint8(1)];
      | TOS_AEBLongTargetBus.vy=OFM_SignalVerification.Object_VY[TOS_AEBLongTargetIndex-uint8(1)];
      | TOS_AEBLongTargetBus.ax=OFM_SignalVerification.Object_AX[TOS_AEBLongTargetIndex-uint8(1)];
      | TOS_AEBLongTargetBus.ay=OFM_SignalVerification.Object_AY[TOS_AEBLongTargetIndex-uint8(1)];
      | TOS_AEBLongTargetBus.dxVariance=OFM_SignalVerification.Object_Std_DX[TOS_AEBLongTargetIndex-uint8(1)];
      | TOS_AEBLongTargetBus.dyVariance=OFM_SignalVerification.Object_Std_DY[TOS_AEBLongTargetIndex-uint8(1)];
      | TOS_AEBLongTargetBus.vxVariance=OFM_SignalVerification.Object_Std_VX[TOS_AEBLongTargetIndex-uint8(1)];
      | TOS_AEBLongTargetBus.vyVariance=OFM_SignalVerification.Object_Std_VY[TOS_AEBLongTargetIndex-uint8(1)];
      | TOS_AEBLongTargetBus.axVariance=OFM_SignalVerification.Object_Std_AX[TOS_AEBLongTargetIndex-uint8(1)];
      | TOS_AEBLongTargetBus.ayVariance=OFM_SignalVerification.Object_Std_AY[TOS_AEBLongTargetIndex-uint8(1)];
      | TOS_AEBLongTargetBus.ObjectLengthVar=OFM_SignalVerification.Object_Std_Length[TOS_AEBLongTargetIndex-uint8(1)];
      | TOS_AEBLongTargetBus.ObjectWidthVar=OFM_SignalVerification.Object_Std_Width[TOS_AEBLongTargetIndex-uint8(1)];
      | TOS_AEBLongTargetBus.ObjectYawAngleVar=OFM_SignalVerification.Object_Std_HeadingAngle[TOS_AEBLongTargetIndex-uint8(1)];
      | TOS_AEBLongTargetBus.ObjectTypeProb=OFM_SignalVerification.Object_Type_Prob[TOS_AEBLongTargetIndex-uint8(1)];
      | TOS_AEBLongTargetBus.ObjectMovingStateProb= single(0);
      | TOS_AEBLongTargetBus.ObjectMovingOrientationProb= single(0);
      | TOS_AEBLongTargetBus.ObjectExistProb=OFM_SignalVerification.Object_ExistProb[TOS_AEBLongTargetIndex-uint8(1)];
      | TOS_AEBLongTargetBus.ObjectIsObstacleProb=OFM_SignalVerification.Object_ObstacleProb[TOS_AEBLongTargetIndex-uint8(1)];
      | TOS_AEBLongTargetBus.ObjectRCS= single(0);
      | TOS_AEBLongTargetBus.ObjectMeasurementStatus= single(0);
      | TOS_AEBLongTargetBus.ObjectLifeCycle=OFM_SignalVerification.Object_Age[TOS_AEBLongTargetIndex-uint8(1)];
      | TOS_AEBLongTargetBus.dyObject2Center=TOS_AddAttributes.PP_ObjectToCenterLine_dy[TOS_AEBLongTargetIndex-uint8(1)];
      | TOS_AEBLongTargetBus.dyEgo2Center=TOS_AddAttributes.PP_EgoVehCenterLine_dy[TOS_AEBLongTargetIndex-uint8(1)];
      | TOS_AEBLongTargetBus.ObjUpdate=false;
      | }
  (junction 5) -> (junction 7)
  (junction 7) -> (junction 11)
  data: OFM_SignalVerification input Bus: OFM_OBJ_BUS; TOS_AddAttributes input Bus: TOS_AddAttributes_BUS; TOS_AEBLongTargetMovingDir input uint8; TOS_AEBLongTargetIndex input uint8; TOS_AEBLongTargetBus output Bus: TOS_AEB_LONOBJ_BUS

== stateflow chart PubIfDecisionTOS_MDL/TOS_20201112/TOS_2012080320/TOS/AEB/TOS_AEBLong/AEBLong_Confirm/AEBLong/AEBLong_TrgConfirm/AEBLongTrgJudg/TOS_AEBLong_ObjFusType/Subsystem/TOS_ObjMovStateCfmFlow1 ==
  note: TOS_ObjMovStateCfm Coding:
      | 0: Object default moving state
      | 1：Object had been moving
      | 2: Object is moving
  (default) -> (junction 1)
  (junction 1) -> (junction 3) [order 1] : [Target_ID_K1 ~=C_TOS_OFMObjIDInvilad_Val&&...
      | Target_ID_K2 ~= C_TOS_OFMObjIDInvilad_Val]
  (junction 1) -> (junction 38) [order 2] : {
      |   TOS_ObjMovStateCfm = uint8(0);
      | }
  (junction 3) -> (junction 5)
  (junction 5) -> (junction 7) [order 1] : [Target_ID_K1 ==Target_ID_K2]
  (junction 5) -> (junction 35) [order 2] : {
      |   TOS_ObjMovStateCfm =uint8(0);
      | }
  (junction 7) -> (junction 9)
  (junction 9) -> (junction 11) [order 1] : [ObjectID ==Target_ID_K1]
  (junction 9) -> (junction 29) [order 2] : {
      |   TOS_ObjMovStateCfm = uint8(0);
      | }
  (junction 11) -> (junction 13)
  (junction 13) -> (junction 15) [order 1] : [(Target_MovState_K2 == ObjectMovingState_E.Moving||...
      | Target_MovState_K2 == ObjectMovingState_E.Stopped)&&...
      | (Target_MovState_K1 == ObjectMovingState_E.Moving||...
      | Target_MovState_K1 == ObjectMovingState_E.Stopped)||...
      |   TOS_ObjMovStateCfm == uint8(1)]
  (junction 13) -> (junction 52) [order 2]
  (junction 15) -> (junction 58) : {
      |   TOS_ObjMovStateCfm = uint8(1);
      | }
  (junction 52) -> (junction 23) [order 1] : [ObjMovState == OFM_OBJ_MOVINGSTATE_E.STOPPED||...
      | ObjMovState == OFM_OBJ_MOVINGSTATE_E.MOVING]
  (junction 52) -> (junction 27) [order 2] : {
      |   TOS_ObjMovStateCfm = uint8(0);
      | }
  (junction 23) -> (junction 54) : {
      |   TOS_ObjMovStateCfm = uint8(2);
      | }
  (junction 35) -> (junction 38)
  (junction 29) -> (junction 35)
  (junction 27) -> (junction 29)
  (junction 54) -> (junction 27)
  (junction 58) -> (junction 54)
  (junction 38) -> (junction 41)
  data: Target_ID_K1 input uint8; Target_ID_K2 input uint8; Target_MovState_K1 input Enum: ObjectMovingState_E; Target_MovState_K2 input Enum: ObjectMovingState_E; ObjMovState input Enum: OFM_OBJ_MOVINGSTATE_E; ObjectID input uint8; TOS_ObjMovStateCfm output uint8; C_TOS_OFMObjIDInvilad_Val parameter uint8

== stateflow chart PubIfDecisionTOS_MDL/TOS_20201112/TOS_2012080320/TOS/AEB/TOS_AEBLong/AEBLong_Confirm/AEBLong/AEBLong_TrgConfirm/AEBLongTrgJudg/TOS_AEBLong_TargetMovingDir/Subsystem/TOS_ObjMovStateCfmFlow ==
  note: TOS_ObjMovStateCfm Coding:
      | 0: Object default moving state
      | 1：Object had been moving
      | 2: Object had been Stopped
  (default) -> (junction 1)
  (junction 1) -> (junction 3) [order 1] : [Target_ID_K1 ~=C_TOS_OFMObjIDInvilad_Val&&...
      | Target_ID_K2 ~= C_TOS_OFMObjIDInvilad_Val]
  (junction 1) -> (junction 38) [order 2] : {
      |   TOS_ObjMovStateCfm = uint8(0);
      | }
  (junction 3) -> (junction 5)
  (junction 5) -> (junction 7) [order 1] : [Target_ID_K1 ==Target_ID_K2]
  (junction 5) -> (junction 35) [order 2] : {
      |   TOS_ObjMovStateCfm =uint8(0);
      | }
  (junction 7) -> (junction 9)
  (junction 9) -> (junction 11) [order 1] : [ObjectID ==Target_ID_K1]
  (junction 9) -> (junction 29) [order 2] : {
      |   TOS_ObjMovStateCfm = uint8(0);
      | }
  (junction 11) -> (junction 13)
  (junction 13) -> (junction 15) [order 1] : [(((Target_MovState_K2 == ObjectMovingState_E.Moving||...
      | Target_MovState_K2 == ObjectMovingState_E.Stopped)||...
      | (Target_MovState_K1 == ObjectMovingState_E.Moving||...
      | Target_MovState_K1 == ObjectMovingState_E.Stopped))&&...
      | (ObjMovState == OFM_OBJ_MOVINGSTATE_E.STATIONARY||...
      | ObjMovState == OFM_OBJ_MOVINGSTATE_E.INVALID||...
      | ObjMovState ==OFM_OBJ_MOVINGSTATE_E.UNKNOWN))||...
      | TOS_ObjMovStateCfm == uint8(1)||...
      | TOS_ObjMovStateCfm == uint8(2)]
  (junction 13) -> (junction 52) [order 2]
  (junction 15) -> (junction 62)
  (junction 62) -> (junction 64) [order 1] : [Target_MovState_K1 == ObjectMovingState_E.Moving]
  (junction 62) -> (junction 68) [order 2]
  (junction 64) -> (junction 66) : {
      |   TOS_ObjMovStateCfm = uint8(1);
      | }
  (junction 52) -> (junction 27) : {
      |   TOS_ObjMovStateCfm = uint8(0);
      | }
  (junction 68) -> (junction 70) [order 1] : [Target_MovState_K1 == ObjectMovingState_E.Stopped]
  (junction 68) -> (junction 58) [order 2]
  (junction 70) -> (junction 72) : {
      |   TOS_ObjMovStateCfm = uint8(2);
      | }
  (junction 35) -> (junction 38)
  (junction 29) -> (junction 35)
  (junction 27) -> (junction 29)
  (junction 58) -> (junction 27)
  (junction 72) -> (junction 58)
  (junction 66) -> (junction 72)
  (junction 38) -> (junction 41)
  data: Target_ID_K1 input uint8; Target_ID_K2 input uint8; Target_MovState_K1 input Enum: ObjectMovingState_E; Target_MovState_K2 input Enum: ObjectMovingState_E; ObjMovState input Enum: OFM_OBJ_MOVINGSTATE_E; ObjectID input uint8; TOS_ObjMovStateCfm output uint8; C_TOS_OFMObjIDInvilad_Val parameter uint8

== stateflow chart PubIfDecisionTOS_MDL/TOS_20201112/TOS_2012080320/TOS/AEB/TOS_AEBLong/AEBLong_Target_PreJudge/AEBLONG_Target_PreFilt/AEBLONG_TargetPreCondJudge/AEBLONGTarget_Fence/Chart ==
  (default) -> (junction 1)
  (junction 1) -> (junction 3) [order 1] : [(FR_Confirm == C_TOS_PP_ObjFusType_FR_Confirm_b)&&...
      | ((Obj_MovingState == OFM_OBJ_MOVINGSTATE_E.STATIONARY)||...
      | (Obj_MovingState == OFM_OBJ_MOVINGSTATE_E.INVALID)||...
      | (Obj_MovingState == OFM_OBJ_MOVINGSTATE_E.UNKNOWN))]
  (junction 1) -> (junction 20) [order 2] : {
      |   ObjectisFence_Flag =false;
      | }
  (junction 3) -> (junction 5)
  (junction 5) -> (junction 35) [order 1] : [Object_ObstacleProb < single(0.85)]
  (junction 5) -> (junction 17) [order 2] : {
      |   ObjectisFence_Flag =false;
      | }
  (junction 35) -> (junction 37)
  (junction 37) -> (junction 39) [order 1] : [abs(Object_DY) < single(1.45) ]
  (junction 37) -> (junction 41) [order 2] : {
      |   ObjectisFence_Flag = true;
      | }
  (junction 39) -> (junction 15) : {
      |   ObjectisFence_Flag = false;
      | }
  (junction 17) -> (junction 20)
  (junction 41) -> (junction 17)
  (junction 15) -> (junction 41)
  (junction 20) -> (junction 23)
  data: FR_Confirm input boolean; Obj_MovingState input Enum: OFM_OBJ_MOVINGSTATE_E; ObjectisFence_Flag output boolean; Object_ObstacleProb input single; Object_DY input single; C_TOS_PP_ObjFusType_FR_Confirm_b parameter

== matlab function PubIfDecisionTOS_MDL/TOS_20201112/TOS_2012080320/TOS/AEB/TOS_AEBLong/MATLAB Function1 ==
  data: Object_Dx input; Object_ID input; Dx1stNearestObjIndex output; Dx1stNearestObjID output; Dx2edNearestObjIndex output; Dx2edNearestObjID output; ConditionJudge input; TargetFusionTypeFlag input; Object_Num input

%%%%ObjDisIndex按Dx从小到大的总排序
%%%%%%%%ObjectID按Dx从小到大的总排序
function [Dx1stNearestObjIndex,Dx1stNearestObjID,Dx2edNearestObjIndex,Dx2edNearestObjID]   = MinMax(Object_Dx,Object_ID,ConditionJudge,TargetFusionTypeFlag,Object_Num)
Dx = Object_Dx;
ID = Object_ID;
for i=int32(1):int32(Object_Num)
    
    if (ID(i) == uint8(0))||(ConditionJudge(i) == false)||(Dx(i) < single(0))||(TargetFusionTypeFlag(i) == false)%%%%%本车道/前方/非0目标
       Dx(i) = single(255);
    end
end

[MinDx1st,MinIndex1st] = min(Dx);
if (MinDx1st > single(250))
   Dx1stNearestObjIndex = uint8(0);
   Dx1stNearestObjID = uint8(0); 
   Dx2edNearestObjIndex = uint8(0);
   Dx2edNearestObjID = uint8(0);
else
    Dx(MinIndex1st) = single(255);
    [MinDx2ed,MinIndex2ed] = min(Dx);
    Dx1stNearestObjIndex = uint8(MinIndex1st);
   Dx1stNearestObjID = uint8(ID(MinIndex1st)); 
   
   if (MinDx2ed > single(250))
     Dx2edNearestObjIndex = uint8(0);
     Dx2edNearestObjID = uint8(0);
   else
     Dx2edNearestObjIndex = uint8(MinIndex2ed);
     Dx2edNearestObjID = uint8(ID(MinIndex2ed));
   end
   

end
end

== matlab function PubIfDecisionTOS_MDL/TOS_20201112/TOS_2012080320/TOS/AEB/TOS_AEBLong/MATLAB Function2 ==
  data: Object_Dx input; Object_ID input; Dx1stNearestObjIndex output; Dx2edNearestObjIndex output; Dx1stNearestObjID output; Dx2edNearestObjID output; ConditionJudge input; TOS_ACC_P0_P1_TargetPreFiltFlag input; Object_Num input; Target_ID_K1 input

%%%%ObjDisIndex按Dx从小到大的总排序
%%%%%%%%ObjectID按Dx从小到大的总排序
function [Dx1stNearestObjIndex,Dx2edNearestObjIndex,Dx1stNearestObjID,Dx2edNearestObjID]   = MinMax(Object_Dx,Object_ID,ConditionJudge,TOS_ACC_P0_P1_TargetPreFiltFlag, Object_Num, Target_ID_K1)
Dx = Object_Dx;
ID = Object_ID;
for i=int32(1):int32(Object_Num)
    
    if (ID(i) == uint8(0))||(ConditionJudge(i) == false)||...
            (Dx(i) < single(0))||(TOS_ACC_P0_P1_TargetPreFiltFlag(i) == false)%%%%%本车道/前方/非0目标
        
       Dx(i) = single(255);
    end
    
    if (Target_ID_K1~=uint8(0))&&(ID(Target_ID_K1)~=uint8(0))&&(i~=Target_ID_K1)
        
        if(abs(Dx(i)- Dx(Target_ID_K1))<single(2))
        
           Dx(i) = single(255);
       
        end
    end
    
    
end

[MinDx1st,MinIndex1st] = min(Dx);
if (MinDx1st > single(250))
   Dx1stNearestObjIndex = uint8(0);
   Dx1stNearestObjID = uint8(0); 
   Dx2edNearestObjIndex = uint8(0);
   Dx2edNearestObjID = uint8(0);
else
    Dx(MinIndex1st) = single(255);
    [MinDx2ed,MinIndex2ed] = min(Dx);
    Dx1stNearestObjIndex = uint8(MinIndex1st);
   Dx1stNearestObjID = uint8(ID(MinIndex1st)); 
   
   if (MinDx2ed > single(250))
     Dx2edNearestObjIndex = uint8(0);
     Dx2edNearestObjID = uint8(0);
   else
     Dx2edNearestObjIndex = uint8(MinIndex2ed);
     Dx2edNearestObjID = uint8(ID(MinIndex2ed));
   end
   

end
end

== stateflow chart PubIfDecisionTOS_MDL/TOS_20201112/TOS_2012080320/TOS/LC_LCKie_ELK/ELK_TargetInfor/TOS_ELKTargetInfor ==
  (default) -> (junction 168) : {i = uint8(1);}
  (junction 168) -> (junction 174) [order 1] : [i <= P_TOS_ELKTargetNum_Val]
  (junction 176) -> (junction 168) : {i=i+uint8(1);}
  (junction 168) -> (junction 171) [order 2]
  (junction 174) -> (junction 176) : {
      | TOS_ELKTargetInfor.Object_Fus_Type(i) = uint8(0);
      | TOS_ELKTargetInfor.Object_ID(i) = uint8(0);
      | TOS_ELKTargetInfor.Object_Type(i) = uint8(0);
      | TOS_ELKTargetInfor.Object_Length(i) = single(0);
      | TOS_ELKTargetInfor.Object_Width(i) = single(0);
      | TOS_ELKTargetInfor.Object_Hight(i) =single(0);
      | TOS_ELKTargetInfor.Object_HeadingAngle(i) =single(0);
      | TOS_ELKTargetInfor.Object_YawAngle(i) = single(0);
      | TOS_ELKTargetInfor.Object_MovingState(i) = uint8(0);
      | TOS_ELKTargetInfor.Object_Orientation(i) = uint8(0);
      | TOS_ELKTargetInfor.Object_DX(i) = single(0);
      | TOS_ELKTargetInfor.Object_DY(i) = single(0);
      | TOS_ELKTargetInfor.Object_VX(i) = single(0);
      | TOS_ELKTargetInfor.Object_VY(i) = single(0);
      | TOS_ELKTargetInfor.Object_Std_AX(i) = single(0);
      | TOS_ELKTargetInfor.Object_Std_AY(i) = single(0);
      | TOS_ELKTargetInfor.Object_Std_DX(i) = single(0);
      | TOS_ELKTargetInfor.Object_Std_DY(i) = single(0);
      | TOS_ELKTargetInfor.Object_Std_VX(i) = single(0);
      | TOS_ELKTargetInfor.Object_Std_VY(i) = single(0);
      | TOS_ELKTargetInfor.Object_AX(i) = single(0);
      | TOS_ELKTargetInfor.Object_AY(i) = single(0);
      | TOS_ELKTargetInfor.Object_Std_Length(i) = single(0);
      | TOS_ELKTargetInfor.Object_Std_Width(i) = single(0);
      | TOS_ELKTargetInfor.Object_Std_HeadingAngle(i) = single(0);
      | TOS_ELKTargetInfor.Object_Type_Prob(i) = single(0);
      | TOS_ELKTargetInfor.Object_ExistProb(i) = single(0);
      | TOS_ELKTargetInfor.Object_ObstacleProb(i) = single(0);
      | TOS_ELKTargetInfor.Object_Age(i) = uint16(0);
      | TOS_ELKTargetInfor.CurrentLane_Prob(i) = single(0);
      | TOS_ELKTargetInfor.LeftLane_Prob(i) = single(0);
      | TOS_ELKTargetInfor.RightLane_Prob(i) = single(0);
      | TOS_ELKTargetInfor.ObjectIn_Lane(i) = uint8(0);
      | }
  (junction 171) -> (junction 155)
  (junction 155) -> (junction 159) : {i=uint8(1);
      | TargetIndex = uint8(0);}
  (junction 159) -> (junction 162) [order 1] : [i <= P_TOS_ELKTargetNum_Val]
  (junction 161) -> (junction 159) : {i=i+uint8(1);}
  (junction 159) -> (junction 158) [order 2]
  (junction 162) -> (junction 181)
  (junction 181) -> (junction 166) [order 1] : [TOS_HWA_TargetIndexVector(i)~=uint8(0)]
  (junction 181) -> (junction 178) [order 2]
  (junction 166) -> (junction 184) : {TargetIndex=TOS_HWA_TargetIndexVector(i);
      | TOS_ELKTargetInfor.Object_Fus_Type(i) = OFM_SignalVerification.Object_Fus_Type(TargetIndex);
      | TOS_ELKTargetInfor.Object_ID(i) = OFM_SignalVerification.Object_ID(TargetIndex);
      | TOS_ELKTargetInfor.Object_Type(i) = OFM_SignalVerification.Object_Type(TargetIndex);
      | TOS_ELKTargetInfor.Object_Length(i) = OFM_SignalVerification.Object_Length(TargetIndex);
      | TOS_ELKTargetInfor.Object_Width(i) = OFM_SignalVerification.Object_Width(TargetIndex);
      | TOS_ELKTargetInfor.Object_Hight(i) = OFM_SignalVerification.Object_Hight(TargetIndex);
      | TOS_ELKTargetInfor.Object_HeadingAngle(i) = OFM_SignalVerification.Object_HeadingAngle(TargetIndex);
      | TOS_ELKTargetInfor.Object_YawAngle(i) = OFM_SignalVerification.Object_YawAngle(TargetIndex);
      | TOS_ELKTargetInfor.Object_MovingState(i) = TOS_AddAttributes.PP_MovingStateSignalProcessing(TargetIndex);
      | TOS_ELKTargetInfor.Object_Orientation(i) = TOS_AddAttributes.PP_ObjMovingDirSignalProcessing(TargetIndex);
      | TOS_ELKTargetInfor.Object_DX(i) = OFM_SignalVerification.Object_DX(TargetIndex);
      | TOS_ELKTargetInfor.Object_DY(i) = OFM_SignalVerification.Object_DY(TargetIndex);
      | TOS_ELKTargetInfor.Object_VX(i) = OFM_SignalVerification.Object_VX(TargetIndex);
      | TOS_ELKTargetInfor.Object_VY(i) = OFM_SignalVerification.Object_VY(TargetIndex);
      | TOS_ELKTargetInfor.Object_Std_AX(i) = OFM_SignalVerification.Object_Std_AX(TargetIndex);
      | TOS_ELKTargetInfor.Object_Std_AY(i) = OFM_SignalVerification.Object_Std_AY(TargetIndex);
      | TOS_ELKTargetInfor.Object_Std_DX(i) = OFM_SignalVerification.Object_Std_DX(TargetIndex);
      | TOS_ELKTargetInfor.Object_Std_DY(i) = OFM_SignalVerification.Object_Std_DY(TargetIndex);
      | TOS_ELKTargetInfor.Object_Std_VX(i) = OFM_SignalVerification.Object_Std_VX(TargetIndex);
      | TOS_ELKTargetInfor.Object_Std_VY(i) = OFM_SignalVerification.Object_Std_VY(TargetIndex);
      | TOS_ELKTargetInfor.Object_AX(i) = OFM_SignalVerification.Object_AX(TargetIndex);
      | TOS_ELKTargetInfor.Object_AY(i) = OFM_SignalVerification.Object_AY(TargetIndex);
      | TOS_ELKTargetInfor.Object_Std_Length(i) = OFM_SignalVerification.Object_Std_Length(TargetIndex);
      | TOS_ELKTargetInfor.Object_Std_Width(i) = OFM_SignalVerification.Object_Std_Width(TargetIndex);
      | TOS_ELKTargetInfor.Object_Std_HeadingAngle(i) = OFM_SignalVerification.Object_Std_HeadingAngle(TargetIndex);
      | TOS_ELKTargetInfor.Object_Type_Prob(i) = OFM_SignalVerification.Object_Type_Prob(TargetIndex);
      | TOS_ELKTargetInfor.Object_ExistProb(i) = OFM_SignalVerification.Object_ExistProb(TargetIndex);
      | TOS_ELKTargetInfor.Object_ObstacleProb(i) = OFM_SignalVerification.Object_ObstacleProb(TargetIndex);
      | TOS_ELKTargetInfor.Object_Age(i) = OFM_SignalVerification.Object_Age(TargetIndex);
      | TOS_ELKTargetInfor.CurrentLane_Prob(i) = TOS_ProbInLaneCalculat.PIL_CurrentLaneProb(TargetIndex);
      | TOS_ELKTargetInfor.LeftLane_Prob(i) = TOS_ProbInLaneCalculat.PIL_LeftLaneProb(TargetIndex);
      | TOS_ELKTargetInfor.RightLane_Prob(i) = TOS_ProbInLaneCalculat.PIL_RightLaneProb(TargetIndex);
      | TOS_ELKTargetInfor.ObjectIn_Lane(i) = ObjectIn_Lane_b(i);
      | }
  (junction 184) -> (junction 178)
  (junction 178) -> (junction 161)
  (junction 158) -> (junction 165)
  data: OFM_SignalVerification input Bus: OFM_OBJ_BUS; TOS_AddAttributes input Bus: TOS_AddAttributes_BUS; TOS_ProbInLaneCalculat input Bus: PIL_ProbInLaneCalculat_BUS; ObjectIn_Lane_b input uint8; TOS_HWA_TargetIndexVector input size=11; TOS_ELKTargetInfor output Bus: TOS_ELK_BUS size=1 =0; P_TOS_ELKTargetNum_Val parameter uint8 size=1; TargetIndex local uint8 size=1; i local uint8 size=1
